simulink model "ver_ondinhas"  (R2025a)
settings: Solver=VariableStepAuto  StartTime=0.0  StopTime=10.0  MaxStep=0.01  RelTol=1e-3
settings Model: Creator=joasb  LastModifiedBy=joasb

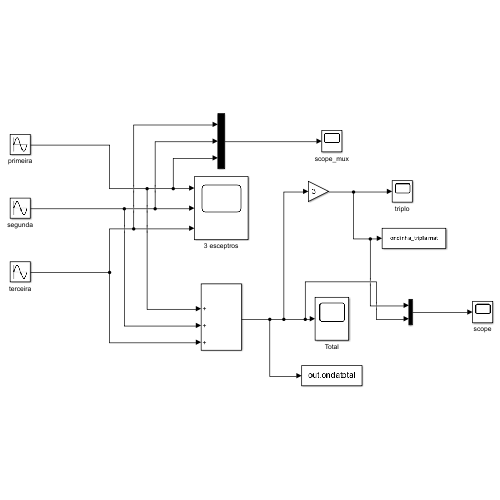
[thumbnail: Simulink's stored preview of the top-level diagram]
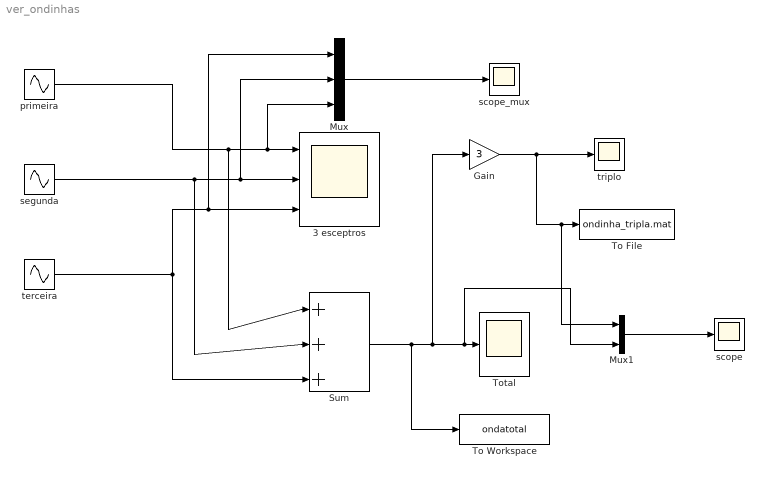
== system ver_ondinhas ==
  3 esceptros : Scope  NumInputPorts=3
      settings: ActiveDisplayYMinimum=-1.2499967500526621  ActiveDisplayYMaximum=1.2499992865967788
  Gain : Gain  Gain=3
  Mux : Mux  Inputs=3
  Mux1 : Mux  Inputs=2
  Sum : Sum  Inputs=|+++
  To File : ToFile  Filename=ondinha_tripla.mat  MatrixName=ondinha  SaveFormat=Timeseries
  To Workspace : ToWorkspace  VariableName=ondatotal  SaveFormat=Timeseries  SampleTime=-1
  Total : Scope
      settings: ActiveDisplayYMinimum=-3.4400175950066787  ActiveDisplayYMaximum=3.4399800198065611
  primeira : Sin  SampleTime=0
  scope : Scope
      settings: ActiveDisplayYMinimum=-10.320052785020037  ActiveDisplayYMaximum=10.319940059419684  DataLoggingVariableName=ScopeData4
  scope_mux : Scope
      settings: ActiveDisplayYMinimum=-1  ActiveDisplayYMaximum=1  DataLoggingVariableName=ScopeData2
  segunda : Sin  Frequency=5  SampleTime=0
  terceira : Sin  Frequency=10  SampleTime=0
  triplo : Scope
      settings: ActiveDisplayYMinimum=-10.320052785020037  ActiveDisplayYMaximum=10.319940059419684  DataLoggingVariableName=ScopeData3
  wires:
  primeira/1 -> Sum/1, Mux/3, 3 esceptros/1
  segunda/1 -> Sum/2, Mux/2, 3 esceptros/2
  terceira/1 -> Mux/1, 3 esceptros/3, Sum/3
  Sum/1 -> To Workspace/1, Gain/1, Mux1/2, Total/1
  Mux/1 -> scope_mux/1
  Gain/1 -> Mux1/1, To File/1, triplo/1
  Mux1/1 -> scope/1
